simulink model "ExampleBicycle6DOF"  (Simulink 8.2)
settings: Solver=FixedStepDiscrete  StartTime=0.0  StopTime=inf  FixedStep=0.001  RelTol=1e-3
libraries: rFproPhysicsLib x5
settings Model: Creator=enewton  LastModifiedBy=Akinori
settings RTWCC: SystemTargetFile=rfpro.tlc  MakeCommand="make_rtw OPTS=\"-DRUN_PHYSICS\""  TemplateMakefile=rfpro.tmf  Description=rFpro Target (Run Physics)  ProcessScript=rfpro_make_rtw_hook  TargetLang=C++
settings STFCustomTargetCC: CodeReplacementLibrary=ANSI_C  ModelReferenceCompliant=off  GeneratePreprocessorConditionals=Disable all  CombineOutputUpdateFcns=on  MatFileLogging=on  GRTInterface=off  SystemTargetFile=rfpro.tlc
settings GRTTargetCC: ModelReferenceCompliant=off  ParMdlRefBuildCompliant=off  CompOptLevelCompliant=off  ConcurrentExecutionCompliant=off  CombineOutputUpdateFcns=on  GRTInterface=off

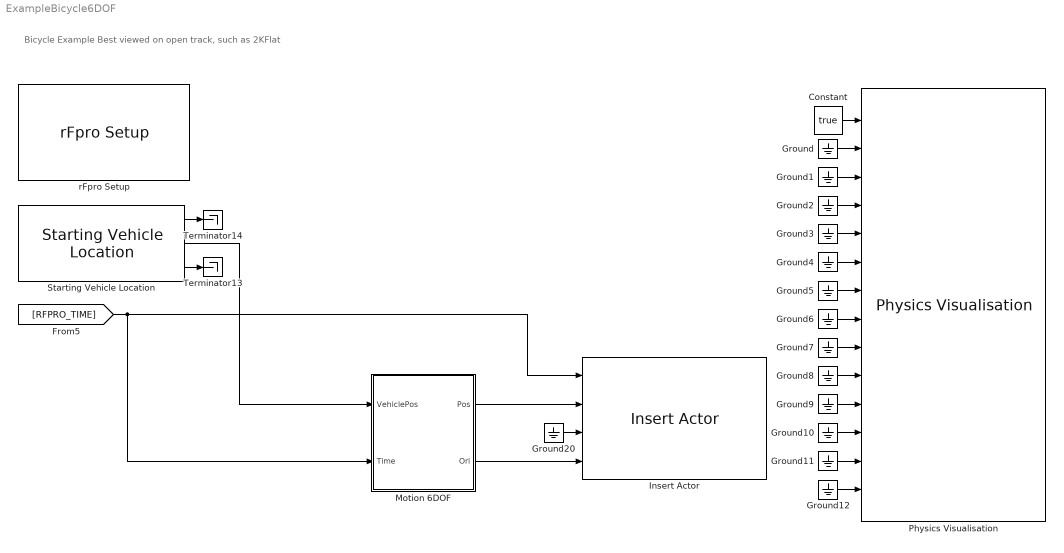
== system ExampleBicycle6DOF ==
  note: Bicycle Example
      | Best viewed on open track, such as 2KFlat
  Constant : Constant  Value=true
  Ground{,1..12,20} (14 alike) : Ground
  Insert Actor : rFproPhysicsLib/Insert Actor  actorType='bike01'  instanceName=''  specialType=Bicycle  doPreLoad=on  headingValid=off  heightValid=on  fixedHeight=0  relHeightFlag=on  orientationValid=on  period=-1  offset=0  useReverseByteOrder=off  rFpro__platform=Remote Model - Default
  Motion 6DOF : Subsystem
  Physics Visualisation : rFproPhysicsLib/Physics Visualisation  PAR_SKIP_INTERNAL_PHYSICS=off  PAR_ACCEL_VALID=off  PAR_ROT_ACCEL_VALID=off  PAR_GEAR_VALID=off  PAR_RPM_VALID=off  PAR_INPUTS_VALID=on  PAR_STEER_TORQUE_VALID=on  PAR_HEADLIGHTS_ON_VALID=off  PAR_WHEEL_POS_VALID=off  PAR_WHEEL_ORI_VALID=off  PAR_TYRE_PARAMS_VALID=off  PAR_WHEEL_ROTATION_VALID=off  PAR_WHEEL_BRAKE_TEMP_VALID=off  PAR_WHEEL_TREAD_TEMP_VALID=off  PAR_WHEEL_AIR_TEMP_VALID=off  period=-1  offset=0  useReverseByteOrder=on  rFpro__platform=Remote Model - Default
  Starting Vehicle Location : rFproPhysicsLib/Starting Vehicle Location  cg_offset=[0, 0, 0]  numPackets=1  rFpro__platform=Remote Model - Default
  Terminator13 : Terminator
  Terminator14 : Terminator
  rFpro Setup : rFproPhysicsLib/rFpro Setup  platform=Remote Model - Default  stopOnSessionEnd=on  usePseudoRealtime=on  syncToRF=on  useReverseByteOrder=off  minIterations=4  maxIterations=1000  ipReceiveAddress='127.0.0.1'  ipReceivePort=11054  receiveSampleTime=-1  ipTransmitAddress='127.0.0.1'  ipTransmitPort=11052  transmitSampleTime=-1  pluginType=RUN_PHYSICS  sysTarget=xpctarget.tlc  templateMakeFile=xpc_default_tmf  makeCommand=make_rtw  buildDesc=xPC target
  wires:
  Starting Vehicle Location/3 -> Terminator13/1
  Starting Vehicle Location/1 -> Terminator14/1
  [RFPRO_TIME] -> Insert Actor/1, Motion 6DOF/2(Time)
  Ground20/1 -> Insert Actor/3
  Starting Vehicle Location/2 -> Motion 6DOF/1(VehiclePos)
  Motion 6DOF/2(Ori) -> Insert Actor/4
  Motion 6DOF/1(Pos) -> Insert Actor/2
  Constant/1 -> Physics Visualisation/1
  Ground/1 -> Physics Visualisation/2
  Ground1/1 -> Physics Visualisation/3
  Ground2/1 -> Physics Visualisation/4
  Ground3/1 -> Physics Visualisation/5
  Ground4/1 -> Physics Visualisation/6
  Ground5/1 -> Physics Visualisation/7
  Ground6/1 -> Physics Visualisation/8
  Ground7/1 -> Physics Visualisation/9
  Ground8/1 -> Physics Visualisation/10
  Ground9/1 -> Physics Visualisation/11
  Ground10/1 -> Physics Visualisation/12
  Ground11/1 -> Physics Visualisation/13
  Ground12/1 -> Physics Visualisation/14

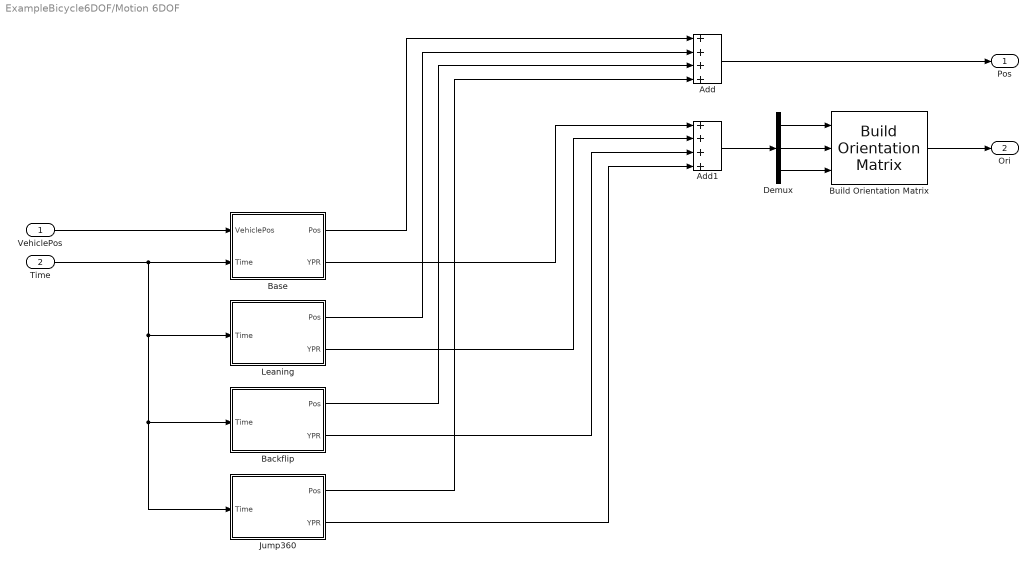
== system ExampleBicycle6DOF/Motion 6DOF ==
  VehiclePos : Inport
  Time : Inport  Port=2
  Add : Sum  Inputs=++++
  Add1 : Sum  Inputs=++++
  Backflip : Subsystem
  Base : Subsystem
  Build Orientation Matrix : rFproPhysicsLib/Build Orientation Matrix  ISOAxes=on  YPROrder=on
  Demux : Demux  Outputs=3
  Jump360 : Subsystem
  Leaning : Subsystem
  Pos : Outport
  Ori : Outport  Port=2
  wires:
  VehiclePos/1 -> Base/1(VehiclePos)
  Time/1 -> Leaning/1(Time), Jump360/1(Time), Backflip/1(Time), Base/2(Time)
  Add/1 -> Pos/1
  Demux/1 -> Build Orientation Matrix/1
  Demux/2 -> Build Orientation Matrix/2
  Demux/3 -> Build Orientation Matrix/3
  Add1/1 -> Demux/1
  Build Orientation Matrix/1 -> Ori/1
  Base/1(Pos) -> Add/1
  Leaning/1(Pos) -> Add/2
  Backflip/1(Pos) -> Add/3
  Jump360/1(Pos) -> Add/4
  Base/2(YPR) -> Add1/1
  Leaning/2(YPR) -> Add1/2
  Backflip/2(YPR) -> Add1/3
  Jump360/2(YPR) -> Add1/4

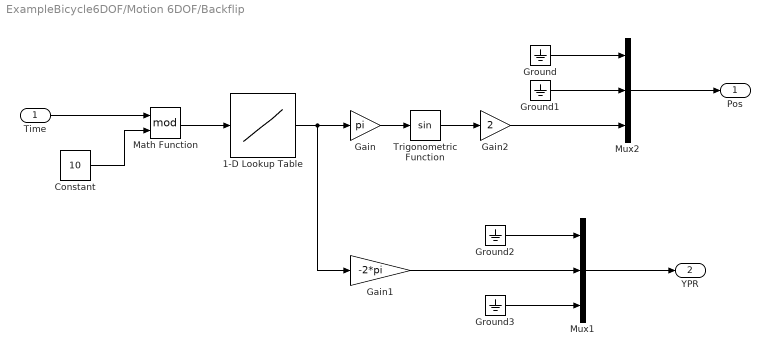
== system ExampleBicycle6DOF/Motion 6DOF/Backflip ==
  Time : Inport
  1-D Lookup Table : Lookup_n-D  NumberOfTableDimensions=1  BreakpointsForDimension1=[0 5 6 10]  Table=[0 0 1 1]  InternalRulePriority=Speed  RndMeth=Simplest  InputSameDT=on
  Constant : Constant  Value=10
  Gain : Gain  Gain=pi
  Gain1 : Gain  Gain=-2*pi
  Gain2 : Gain  Gain=2
  Ground{,1..3} (4 alike) : Ground
  Math Function : Math  Operator=mod  SaturateOnIntegerOverflow=on
  Mux1 : Mux  Inputs=3
  Mux2 : Mux  Inputs=3
  Trigonometric Function : Trigonometry
  Pos : Outport
  YPR : Outport  Port=2
  wires:
  Ground/1 -> Mux2/1
  Ground1/1 -> Mux2/2
  Time/1 -> Math Function/1
  Constant/1 -> Math Function/2
  Math Function/1 -> 1-D Lookup Table/1
  1-D Lookup Table/1 -> Gain1/1, Gain/1
  Gain/1 -> Trigonometric Function/1
  Trigonometric Function/1 -> Gain2/1
  Mux2/1 -> Pos/1
  Mux1/1 -> YPR/1
  Gain2/1 -> Mux2/3
  Ground3/1 -> Mux1/3
  Gain1/1 -> Mux1/2
  Ground2/1 -> Mux1/1

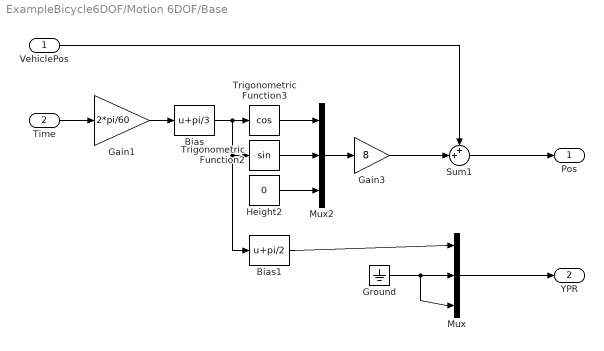
== system ExampleBicycle6DOF/Motion 6DOF/Base ==
  VehiclePos : Inport
  Time : Inport  Port=2
  Bias : Bias  Bias=pi/3
  Bias1 : Bias  Bias=pi/2
  Gain1 : Gain  Gain=2*pi/60
  Gain3 : Gain  Gain=8
  Ground : Ground
  Height2 : Constant  Value=0
  Mux : Mux  Inputs=3
  Mux2 : Mux  Inputs=3
  Sum1 : Sum  Inputs=++|
  Trigonometric Function2 : Trigonometry
  Trigonometric Function3 : Trigonometry  Operator=cos
  Pos : Outport
  YPR : Outport  Port=2
  wires:
  Time/1 -> Gain1/1
  Gain1/1 -> Bias/1
  Bias/1 -> Bias1/1, Trigonometric Function2/1, Trigonometric Function3/1
  Height2/1 -> Mux2/3
  Trigonometric Function2/1 -> Mux2/2
  Trigonometric Function3/1 -> Mux2/1
  Sum1/1 -> Pos/1
  VehiclePos/1 -> Sum1/1
  Mux2/1 -> Gain3/1
  Gain3/1 -> Sum1/2
  Mux/1 -> YPR/1
  Bias1/1 -> Mux/1
  Ground/1 -> Mux/3, Mux/2

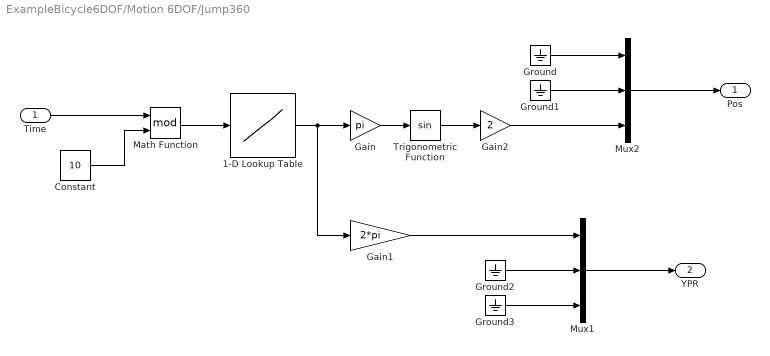
== system ExampleBicycle6DOF/Motion 6DOF/Jump360 ==
  Time : Inport
  1-D Lookup Table : Lookup_n-D  NumberOfTableDimensions=1  BreakpointsForDimension1=[0 7 8 10]  Table=[0 0 1 1]  InternalRulePriority=Speed  RndMeth=Simplest  InputSameDT=on
  Constant : Constant  Value=10
  Gain : Gain  Gain=pi
  Gain1 : Gain  Gain=2*pi
  Gain2 : Gain  Gain=2
  Ground{,1..3} (4 alike) : Ground
  Math Function : Math  Operator=mod  SaturateOnIntegerOverflow=on
  Mux1 : Mux  Inputs=3
  Mux2 : Mux  Inputs=3
  Trigonometric Function : Trigonometry
  Pos : Outport
  YPR : Outport  Port=2
  wires:
  Ground/1 -> Mux2/1
  Ground1/1 -> Mux2/2
  Time/1 -> Math Function/1
  Constant/1 -> Math Function/2
  Math Function/1 -> 1-D Lookup Table/1
  1-D Lookup Table/1 -> Gain1/1, Gain/1
  Gain/1 -> Trigonometric Function/1
  Trigonometric Function/1 -> Gain2/1
  Mux2/1 -> Pos/1
  Mux1/1 -> YPR/1
  Gain2/1 -> Mux2/3
  Ground3/1 -> Mux1/3
  Ground2/1 -> Mux1/2
  Gain1/1 -> Mux1/1

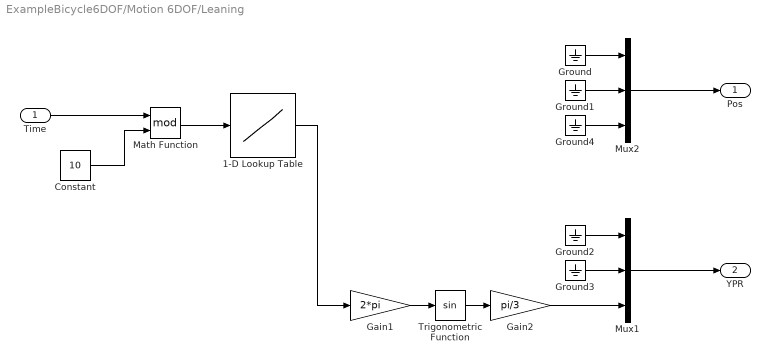
== system ExampleBicycle6DOF/Motion 6DOF/Leaning ==
  Time : Inport
  1-D Lookup Table : Lookup_n-D  NumberOfTableDimensions=1  BreakpointsForDimension1=[0 1 4 10]  Table=[0 0 1 1]  InternalRulePriority=Speed  RndMeth=Simplest  InputSameDT=on
  Constant : Constant  Value=10
  Gain1 : Gain  Gain=2*pi
  Gain2 : Gain  Gain=pi/3
  Ground{,1..4} (5 alike) : Ground
  Math Function : Math  Operator=mod  SaturateOnIntegerOverflow=on
  Mux1 : Mux  Inputs=3
  Mux2 : Mux  Inputs=3
  Trigonometric Function : Trigonometry
  Pos : Outport
  YPR : Outport  Port=2
  wires:
  Ground/1 -> Mux2/1
  Ground1/1 -> Mux2/2
  Time/1 -> Math Function/1
  Constant/1 -> Math Function/2
  Math Function/1 -> 1-D Lookup Table/1
  1-D Lookup Table/1 -> Gain1/1
  Mux2/1 -> Pos/1
  Mux1/1 -> YPR/1
  Ground2/1 -> Mux1/1
  Ground4/1 -> Mux2/3
  Ground3/1 -> Mux1/2
  Gain1/1 -> Trigonometric Function/1
  Trigonometric Function/1 -> Gain2/1
  Gain2/1 -> Mux1/3
